simulink model "simulink_silnik_fuzzy_controller"  (R2023b)
settings: Solver=ode1  StartTime=0.0  StopTime=4  FixedStep=ts  RelTol=1e-3  EnableMultiTasking=on
values from neighbouring files (symbols this model uses):
  ki = x(2)    [f_error_func.m]    (also in f_error_func_v2.m; fuzzy_controller.m = 18.3255)
  kp = x(1)    [f_error_func.m]    (also in f_error_func_v2.m; fuzzy_controller.m = 8.253)
  te = 0.005    [fuzzy_conr.m]    (also in fuzzy_controller.m; opti.m)
  tm = 0.2    [fuzzy_conr.m]    (also in fuzzy_controller.m; opti.m)
settings Model: Creator=j_4k  LastModifiedBy=j_4k
settings DataIOCC: SaveOutput=off  SignalLogging=off  DSMLogging=off  SaveTime=off  ReturnWorkspaceOutputs=off

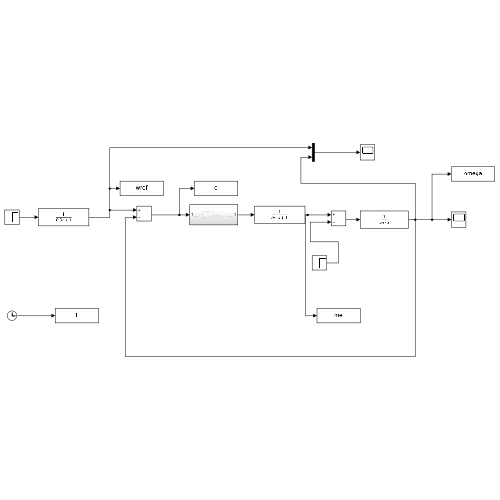
[thumbnail: Simulink's stored preview of the top-level diagram]
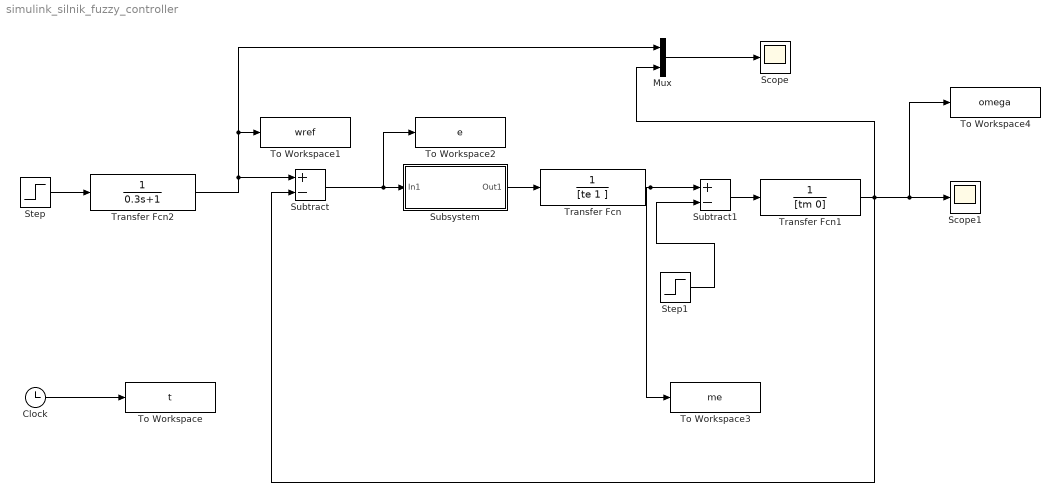
== system simulink_silnik_fuzzy_controller ==
  Clock : Clock
  Mux : Mux  Inputs=2
  Scope : Scope
  Scope1 : Scope
  Step : Step  SampleTime=0
  Step1 : Step  Time=2  SampleTime=0
  Subsystem : Subsystem
  Subtract : Sum  Inputs=+-
  Subtract1 : Sum  Inputs=+-
  To Workspace : ToWorkspace  VariableName=t  SaveFormat=Timeseries  SampleTime=-1
  To Workspace1 : ToWorkspace  VariableName=wref  SaveFormat=Timeseries  SampleTime=-1
  To Workspace2 : ToWorkspace  VariableName=e  SampleTime=-1
  To Workspace3 : ToWorkspace  VariableName=me  SaveFormat=Timeseries  SampleTime=-1
  To Workspace4 : ToWorkspace  VariableName=omega  SaveFormat=Timeseries  SampleTime=-1
  Transfer Fcn : TransferFcn  Denominator=[te 1 ]
  Transfer Fcn1 : TransferFcn  Denominator=[tm 0]
  Transfer Fcn2 : TransferFcn  Denominator=[0.3 1]
  wires:
  Step/1 -> Transfer Fcn2/1
  Subsystem/1(Out1) -> Transfer Fcn/1
  Subtract/1 -> To Workspace2/1, Subsystem/1(In1)
  Step1/1 -> Subtract1/2
  Subtract1/1 -> Transfer Fcn1/1
  Transfer Fcn/1 -> Subtract1/1, To Workspace3/1
  Mux/1 -> Scope/1
  Transfer Fcn1/1 -> Subtract/2, Mux/2, To Workspace4/1, Scope1/1
  Clock/1 -> To Workspace/1
  Transfer Fcn2/1 -> Subtract/1, Mux/1, To Workspace1/1

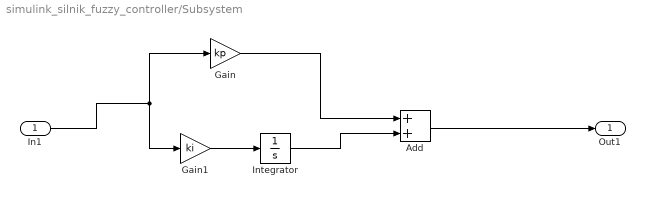
== system simulink_silnik_fuzzy_controller/Subsystem ==
  In1 : Inport
  Add : Sum
  Gain : Gain  Gain=kp
  Gain1 : Gain  Gain=ki
  Integrator : Integrator
  Out1 : Outport
  wires:
  In1/1 -> Gain1/1, Gain/1
  Gain1/1 -> Integrator/1
  Integrator/1 -> Add/2
  Gain/1 -> Add/1
  Add/1 -> Out1/1
